simulink model "Step_8_AdditionalValidation"  (R2020a)
settings: Solver=VariableStepAuto  StartTime=0.0  StopTime=10000  RelTol=1e-3
settings Model: Creator=nnnmmm  LastModifiedBy=nnnmmm

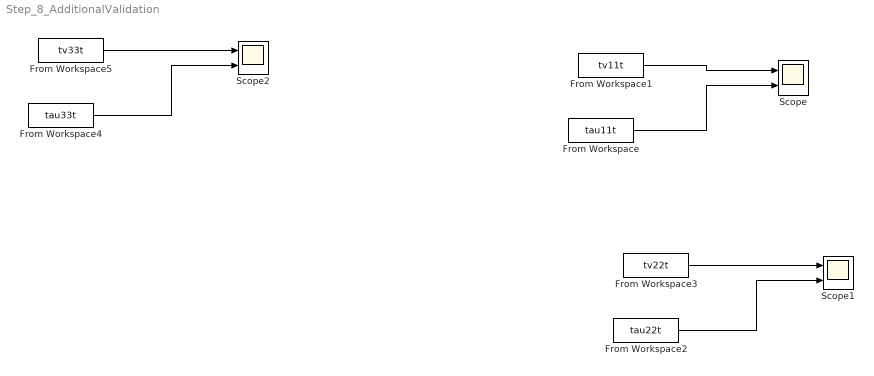
== system Step_8_AdditionalValidation ==
  From Workspace : FromWorkspace  VariableName=tau11t
  From Workspace1 : FromWorkspace  VariableName=tv11t  SampleTime=1/100
  From Workspace2 : FromWorkspace  VariableName=tau22t
  From Workspace3 : FromWorkspace  VariableName=tv22t  SampleTime=1/100
  From Workspace4 : FromWorkspace  VariableName=tau33t
  From Workspace5 : FromWorkspace  VariableName=tv33t  SampleTime=1/100
  Scope : Scope  NumInputPorts=2
  Scope1 : Scope  NumInputPorts=2
  Scope2 : Scope  NumInputPorts=2
  wires:
  From Workspace/1 -> Scope/2
  From Workspace1/1 -> Scope/1
  From Workspace3/1 -> Scope1/1
  From Workspace2/1 -> Scope1/2
  From Workspace4/1 -> Scope2/2
  From Workspace5/1 -> Scope2/1
